simulink model "DTC_clasic1b"  (Simulink 10.2)
settings: Solver=ode3  StartTime=0.0  StopTime=0.5  RelTol=1e-3  EnableMultiTasking=on
libraries: powerlib x7, simulink x1
settings Model: Creator=root  LastModifiedBy=William
settings DataIOCC: LimitDataPoints=on
settings OptimizationCC: ExpressionDepthLimit=2147483647
settings DebuggingCC: SolverPrmCheckMsg=warning  StateNameClashWarn=warning
settings SFSimCC: SimParseCustomCode=off
settings SimscapeCC: SimscapeNormalizeSystem=off

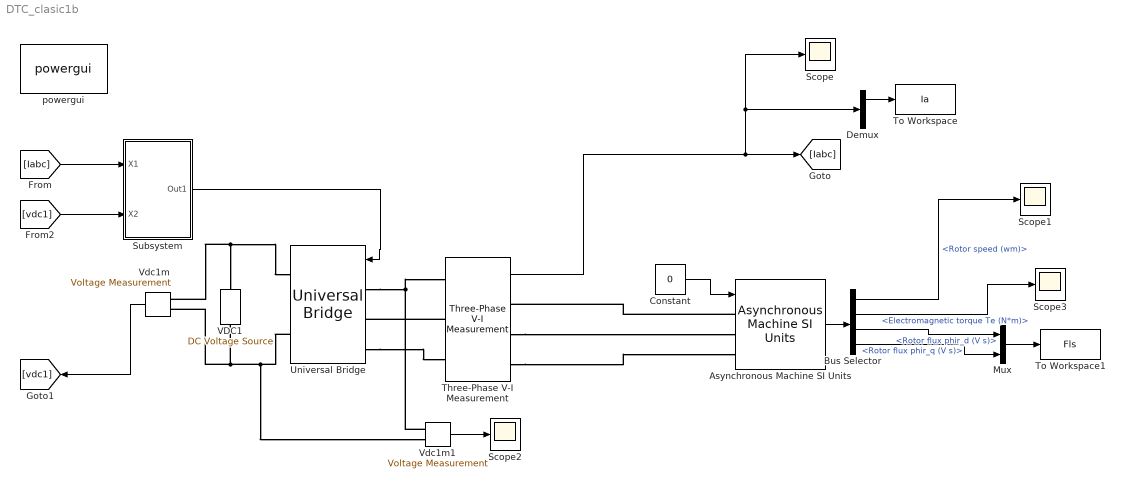
== system DTC_clasic1b ==
  Asynchronous Machine SI Units : powerlib/Machines/Asynchronous Machine SI Units  RotorType=Squirrel-cage  PresetModel=No  MechanicalLoad=Torque Tm  ShowDetailedParameters=on  ReferenceFrame=Stationary  Units=SI  MeasurementBus=off  NominalParameters=[1.845e+04 400 50]  Stator=[0.435 0.002]  Rotor=[0.816 0.002]  Cage1=[0.4155 0.002066]  Cage2=[0.4168 0.0003495]  Lm=0.0693  Mechanical=[0.089 0 2]  PolePairs=2  InitialConditions=[1 0 0 0 0 0 0 0]  SimulateSaturation=off  Saturation=[14.03593122, 27.81365428, 53.79336849, 72.68890987, 97.98006896, 148.6815601, 215.7428561, 302.9841135, 428.7778367 ; 230, 322, 414, 460, 506, 552, 598, 644, 690]  LoadFlowParameters=1492000  TsPowergui=0  TsBlock=-1  IterativeModel=Trapezoidal non iterative  IterativeDiscreteModel=Trapezoidal non iterative  Pmec=1.492e+006
  Bus Selector : BusSelector  OutputSignals=Mechanical.Rotor speed (wm),Mechanical.Electromagnetic torque Te (N*m),Rotor measurements.Rotor flux phir_d (V s),Rotor measurements.Rotor flux phir_q (V s)
  Constant : Constant  Value=0
  Demux : Demux  Outputs=3
  Mux : Mux  Inputs=2
  Scope{,1..3} (4 alike) : Scope
  Subsystem : Subsystem
  Three-Phase V-I Measurement : powerlib/Measurements/Three-Phase V-I Measurement  VoltageMeasurement=no  SetLabelV=off  LabelV=Vabc  Vpu=off  VpuLL=off  CurrentMeasurement=yes  SetLabelI=off  LabelI=Iabc  Ipu=off  Pbase=100e6  Vbase=500e3  OutputType=Complex  PhasorSimulation=off  PSBequivalent=0
  To Workspace : ToWorkspace  VariableName=Ia  SampleTime=-1
  To Workspace1 : ToWorkspace  VariableName=Fls  SampleTime=-1
  Universal Bridge : powerlib/Power Electronics/Universal Bridge  Arms=3  SnubberResistance=1e5  SnubberCapacitance=inf  Device=IGBT / Diodes  Ron=1e-3  Lon=0  ForwardVoltages="[  0  0  ]"  ForwardVoltage=0  GTOparameters=[ 10e-6 , 20e-6 ]  IGBTparameters=[ 1e-6 , 2e-6 ]  Measurements=None  Measurements_2=None  converterType=Rectifier
  VDC1 : powerlib/Electrical Sources/DC Voltage Source  Amplitude=400  Measurements=None
  Vdc1m : powerlib/Measurements/Voltage Measurement  PhasorSimulation=off  OutputType=Complex  PSBequivalent=0
  Vdc1m1 : powerlib/Measurements/Voltage Measurement  PhasorSimulation=off  OutputType=Complex  PSBequivalent=0
  powergui : powerlib/powergui  SimulationMode=Discrete  SampleTime=1e-6  frequency=60  Iterations=50  frequencyindice=0  Pbase=100e6  ErrMax=1e-4  UnitsV=kV  UnitsW=MW  buscounter=0  FunctionMessages=off  echomessages=off  EnableUseOfTLC=off  CurrentSourceSwitches=off  DisableSnubberDevices=off  DisableRonSwitches=off  DisableVfSwitches=off  DisplayEquations=off  AutomaticDiscreteSolvers=off  SolverType=Tustin  Interpol=off  ExternalGateDelay=off  methode=off  Ts=0  x0status=blocks  SPID=off  SwTol=0  HookPort=off  NonlinearTolerance=1e-4  nMaxIteration=100  ContinueOnMaxIteration=off  RestoreLinks=warning  ResistiveCurrentMeasurement=off  Frange=[0:2:500]  Ylog=off  Xlog=on  ShowGrid=off  save=off  variable=ZData  structure=0  ZoomFFT=on  StartTime=0.0  cycles=1  DisplayStyle=1  fundamental=60  FreqAxis=off  MaxFrequency=1000  frequencyindicesteady=1  RmsSteady=1  display=off
  wires:
  Subsystem/1(Out1) -> Universal Bridge/1
  Vdc1m/1 -> [vdc1]
  [Iabc] -> Subsystem/1(X1)
  [vdc1] -> Subsystem/2(X2)
  Three-Phase V-I Measurement/1 -> [Iabc], Scope/1, Demux/1
  Vdc1m1/1 -> Scope2/1
  Demux/1 -> To Workspace/1
  Bus Selector/2 -> Scope3/1  "<Electromagnetic torque Te (N*m)>"
  Asynchronous Machine SI Units/1 -> Bus Selector/1
  Constant/1 -> Asynchronous Machine SI Units/1
  Bus Selector/1 -> Scope1/1  "<Rotor speed (wm)>"
  Bus Selector/3 -> Mux/1  "<Rotor flux phir_d (V s)>"
  Bus Selector/4 -> Mux/2  "<Rotor flux phir_q (V s)>"
  Mux/1 -> To Workspace1/1
  connections:
  Universal Bridge/RConn2 -- Vdc1m1/LConn2 -- VDC1/LConn1 -- Vdc1m/LConn2
  Vdc1m/LConn1 -- VDC1/RConn1 -- Universal Bridge/RConn1
  Vdc1m1/LConn1 -- Universal Bridge/LConn1 -- Three-Phase V-I Measurement/LConn1
  Universal Bridge/LConn3 -- Three-Phase V-I Measurement/LConn3
  Three-Phase V-I Measurement/LConn2 -- Universal Bridge/LConn2
  Three-Phase V-I Measurement/RConn3 -- Asynchronous Machine SI Units/LConn3
  Three-Phase V-I Measurement/RConn2 -- Asynchronous Machine SI Units/LConn2
  Asynchronous Machine SI Units/LConn1 -- Three-Phase V-I Measurement/RConn1

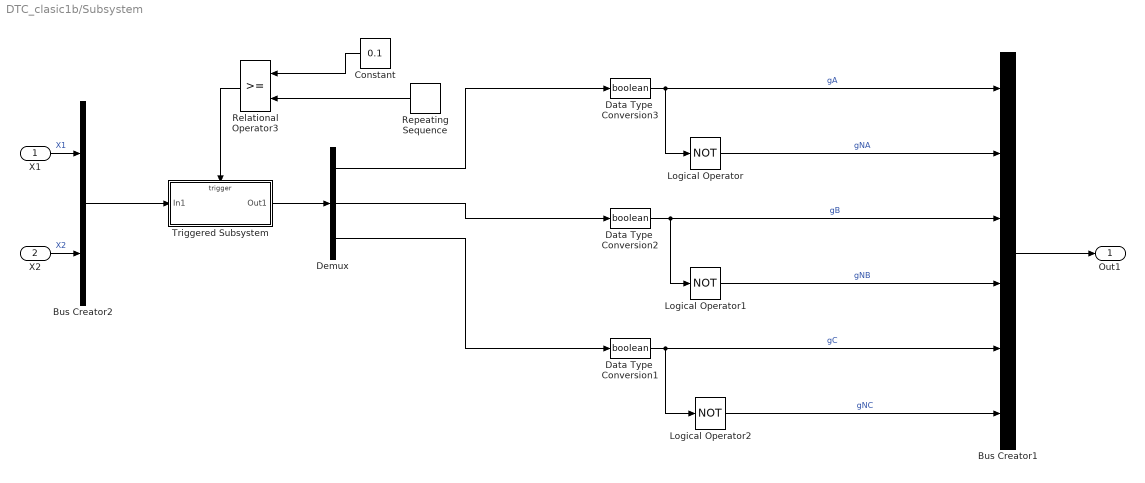
== system DTC_clasic1b/Subsystem ==
  X1 : Inport
  X2 : Inport  Port=2
  Bus Creator1 : BusCreator  Inputs='gA','gNA','gB','gNB','gC','gNC'
  Bus Creator2 : BusCreator  Inputs=2
  Constant : Constant  Value=0.1
  Data Type  Conversion1 : DataTypeConversion  OutDataTypeStr=boolean  SaturateOnIntegerOverflow=on  RndMeth=Zero
  Data Type  Conversion2 : DataTypeConversion  OutDataTypeStr=boolean  SaturateOnIntegerOverflow=on  RndMeth=Zero
  Data Type  Conversion3 : DataTypeConversion  OutDataTypeStr=boolean  SaturateOnIntegerOverflow=on  RndMeth=Zero
  Demux : Demux  Outputs=3
  Logical Operator : Logic  Operator=NOT  AllPortsSameDT=off  OutDataTypeStr=boolean
  Logical Operator1 : Logic  Operator=NOT  AllPortsSameDT=off  OutDataTypeStr=boolean
  Logical Operator2 : Logic  Operator=NOT  AllPortsSameDT=off  OutDataTypeStr=boolean
  Relational Operator3 : RelationalOperator  RndMeth=Nearest  InputSameDT=on
  Repeating Sequence : simulink/Sources/Repeating Sequence  rep_seq_t=[0 50e-6 100e-6]  rep_seq_y=[0 1 0]
  Triggered Subsystem : Subsystem  TreatAsAtomicUnit=on
  Out1 : Outport  VectorParamsAs1DForOutWhenUnconnected=off
  wires:
  Triggered Subsystem/1(Out1) -> Demux/1
  Data Type  Conversion1/1 -> Logical Operator2/1, Bus Creator1/5  "gC"
  Data Type  Conversion2/1 -> Logical Operator1/1, Bus Creator1/3  "gB"
  Bus Creator1/1 -> Out1/1
  Repeating Sequence/1 -> Relational Operator3/2
  Constant/1 -> Relational Operator3/1
  Relational Operator3/1 -> Triggered Subsystem/Trigger
  X1/1 -> Bus Creator2/1  "X1"
  X2/1 -> Bus Creator2/2  "X2"
  Bus Creator2/1 -> Triggered Subsystem/1(In1)
  Logical Operator1/1 -> Bus Creator1/4  "gNB"
  Logical Operator2/1 -> Bus Creator1/6  "gNC"
  Logical Operator/1 -> Bus Creator1/2  "gNA"
  Data Type  Conversion3/1 -> Bus Creator1/1, Logical Operator/1  "gA"
  Demux/1 -> Data Type  Conversion3/1
  Demux/2 -> Data Type  Conversion2/1
  Demux/3 -> Data Type  Conversion1/1

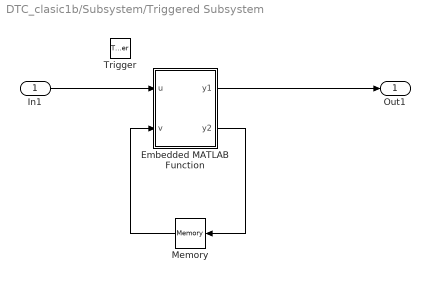
== system DTC_clasic1b/Subsystem/Triggered Subsystem ==
  In1 : Inport  LatchByDelayingOutsideSignal=on
  Trigger : TriggerPort  VariantControl=(inherit)
  Embedded MATLAB Function : MATLAB Function  TreatAsAtomicUnit=on
  Memory : Memory  InitialCondition=[0 0 0 0 ]  InheritSampleTime=on
  Out1 : Outport  VectorParamsAs1DForOutWhenUnconnected=off
  wires:
  In1/1 -> Embedded MATLAB Function/1(u)
  Memory/1 -> Embedded MATLAB Function/2(v)
  Embedded MATLAB Function/1(y1) -> Out1/1
  Embedded MATLAB Function/2(y2) -> Memory/1

== matlab function Subsystem/Triggered Subsystem/Embedded MATLAB Function ==
  data: u input double; y1 output double; v input double; y2 output double
function [y1, y2] = fcn(u, v)
% Direct torque control
%
T2=[ 4 0 2 0 5 0 3 0; %region 1
    5 0 6 0 1 0 2 0; %region 2
    1 0 4 0 3 0 6 0; %region 3
    3 0 5 0 2 0 4 0; %region 4
    2 0 1 0 6 0 5 0; %region 5
    6 0 3 0 4 0 1 0]; %region 6

Rs=0.435;
Lm=69.3e-3;
Ls=Lm+2e-3;
%
Ia=u(1);
Ib=u(2);
Ic=u(3);
Vdc=u(4);

iter=v(1);
trap=v(2);
Fx=v(3);
Fy=v(4);

Fm=sqrt(Fx*Fx+Fy*Fy);
Isx=sqrt(2/3)*(Ia-0.5*Ib-0.5*Ic);
Isy=sqrt(2)/2*(Ib-Ic);
Te=2*Lm/Ls*(Isy*Fx-Isx*Fy);

Fref=0.55;

Teref=12;
Va=0;
Vb=1;
Vc=0;
flag=1;
S1=0;
S2=1;
SW=uint8(0);

if iter<200
    if Fm<0.9*Fref
        flag=0;
    else
        flag=1;
    end
end

if flag==1
    
    % if Fm < 0.7*Fref
    %     Teref=0;
    % end
    rx=0.866025403784*Fm;
    if Fx >= 0
        if Fx>=rx
            S1=1;% region 1
        elseif Fy > 0
            S1=2;% region 2
        else
            S1=6;% region 6
        end
        
    else
        if Fx<=-rx
            S1=4;% region 4
        elseif Fy>0
            S1=3;% region 3
        else
            S1=5;% region 5
        end
    end
    eTe=Teref-Te;
    
    if eTe < -0.1
        S2=1;
    elseif eTe<0.1
        S2=2;
    else
        S2=3;
    end
    
    eF=Fref-Fm;
    if eF > 0
        S2=S2+4;
    end
    
    SW=uint8(T2(S1,S2));
    Va=double(bitand(SW,1));
    Vb=double(bitand(SW,2))/2;
    Vc=double(bitand(SW,4))/4;
end


Vx=sqrt(2/3)*Vdc*(Va-0.5*Vb-0.5*Vc);
Vy=sqrt(2)/2*Vdc*(Vb-Vc);
Isx=sqrt(2/3)*(Ia-0.5*Ib-0.5*Ic);
Isy=sqrt(2)/2*(Ib-Ic);

Fxn=Fx+1e-4*(Vx-Rs*Isx);
Fyn=Fy+1e-4*(Vy-Rs*Isy);
y1 = [Va Vb Vc];
%
y2 = [iter trap Fxn Fyn];
